simulink model "BlueROV2_Exp_Simu_NIF"  (R2023b)
settings: Solver=FixedStepAuto  StartTime=0.0  StopTime=120  FixedStep=dt  RelTol=1e-3
values from neighbouring files (symbols this model uses):
  Af = diag(ti)    [RM_param_AGF.m]
  Ballast_Force = Ballast_Compute(Ballast_Config)    [Integrate.m]    (also in init.m = Ballast_Term(Ballast_Config); init_NIF.m = [0; 0; Ballast_Term; 0]; init_NIF2.m = [0; 0; Ballast_Term; 0]; init_ODE.m)
  dt = 0.1    [Integrate.m]    (also in init.m; init_NIF.m; init_NIF2.m; init_ODE.m)
  Gamma = diag(omega_is)    [RM_param_AGF.m]
  Kd = [155; 355; 8985; 1205; 1205; 1]    [Integrate.m]    (also in init.m = [1; 1; 1; 1; 1; 1]; init_NIF.m; init_NIF2.m; init_ODE.m)
  Ki = [45; 45; 10; 96; 96; 1]    [Integrate.m]    (also in init.m = [1; 1; 1; 1; 1; 1]; init_NIF.m; init_NIF2.m; init_ODE.m)
  Kp = [255; 545; 7095; 2420; 2375; 1]    [Integrate.m]    (also in init.m = [1; 1; 1; 1; 1; 1]; init_NIF.m; init_NIF2.m; init_ODE.m)
  lower_limit = -upper_limit    (= -30)    [Integrate.m]    (also in init.m; init_NIF.m; init_NIF2.m; init_ODE.m)
  Omega = diag(2*omega_is.*zeta_is)    [RM_param_AGF.m]
  Param = BlueROV2_param()    [Integrate.m]    (also in init.m; init_NIF.m; init_NIF2.m; init_ODE.m)
  T_alloc = Thrust_Allocation()    [Integrate.m]    (also in init_NIF.m; init_NIF2.m; init_ODE.m; init_ballast_checking.m)
  T_alloc_ps = pinv(T_alloc' * T_alloc + lambda * eye(size(T_alloc, 2))) * T_alloc'    [Integrate.m]    (also in init_NIF.m; init_NIF2.m; init_ODE.m; init_ballast_checking.m)
  thrust_rate = 5    [Integrate.m]    (also in init.m; init_NIF.m; init_NIF2.m; init_ODE.m)
  upper_limit = 30    [Integrate.m]    (also in init.m; init_NIF.m; init_NIF2.m; init_ODE.m)
undefined symbols (not defined in the file or in its folder): model_val, Phi_ref, Psi_ref, resampled_time, Theta_ref, time_stamps_phi, time_stamps_psi, time_stamps_theta, time_stamps_x, time_stamps_y, time_stamps_z, time_val, X_ref, Y_ref, Z_ref
(part 1 of 2)
settings Model: Creator=goks  LastModifiedBy=HP

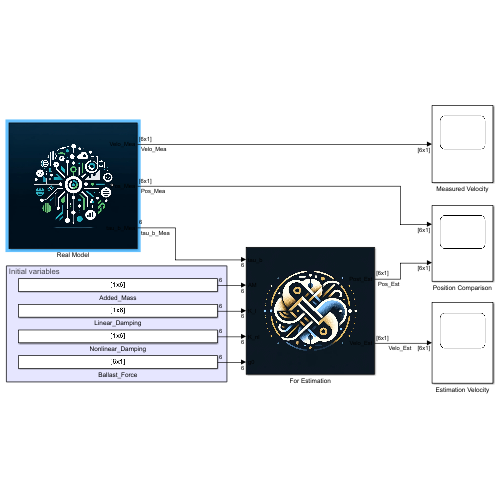
[thumbnail: Simulink's stored preview of the top-level diagram]
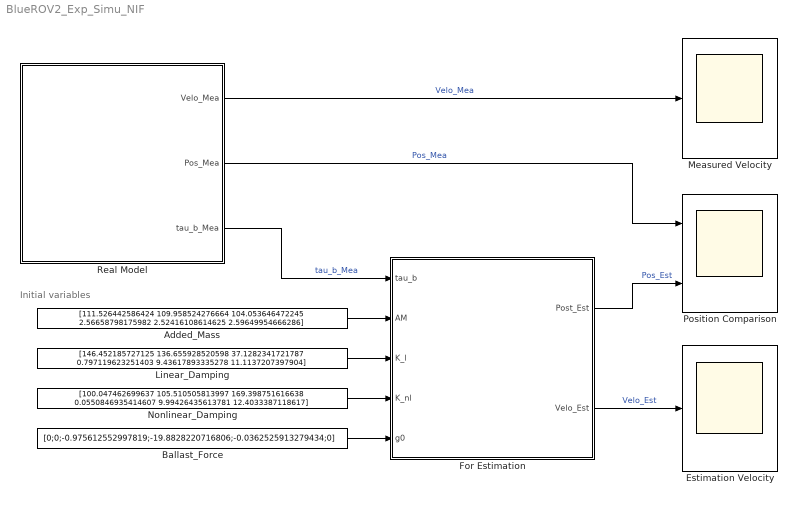
== system BlueROV2_Exp_Simu_NIF ==
  note: Initial variables
  Added_Mass : Constant  Value=[111.526442586424 109.958524276664 104.053646472245 2.56658798175982 2.52416108614625 2.59649954666286]
  Ballast_Force : Constant  Value=[0;0;-0.975612552997819;-19.8828220716806;-0.0362525913279434;0]
  Estimation Velocity : Scope
  For Estimation : Subsystem
      mask Display: image('estimated.jpg');
  Linear_Damping : Constant  Value=[146.452185727125 136.655928520598 37.1282341721787 0.797119623251403 9.43617893335278 11.1137207397904]
  Measured Velocity : Scope
  Nonlinear_Damping : Constant  Value=[100.047462699637 105.510505813997 169.398751616638 0.0550846935414607 9.99426435613781 12.4033387118617]
  Position Comparison : Scope  NumInputPorts=2
  Real Model : Subsystem
      mask Display: image('measured.jpg');
  wires:
  Real Model/1(Velo_Mea) -> Measured Velocity/1  "Velo_Mea"
  For Estimation/2(Velo_Est) -> Estimation Velocity/1  "Velo_Est"
  Added_Mass/1 -> For Estimation/2(AM)
  Linear_Damping/1 -> For Estimation/3(K_l)
  Nonlinear_Damping/1 -> For Estimation/4(K_nl)
  Real Model/2(Pos_Mea) -> Position Comparison/1  "Pos_Mea"
  For Estimation/1(Post_Est) -> Position Comparison/2  "Pos_Est"
  Real Model/3(tau_b_Mea) -> For Estimation/1(tau_b)  "tau_b_Mea"
  Ballast_Force/1 -> For Estimation/5(g0)

== system BlueROV2_Exp_Simu_NIF/For Estimation ==
  note: NIF Input
  tau_b : Inport
  AM : Inport  Port=2
  K_l : Inport  Port=3
  K_nl : Inport  Port=4
  g0 : Inport  Port=5
  BlueROV2 : Subsystem
      mask DialogControl DescTextVar Prompt: %<BlueROV2>
      mask Display: image('heavy-bluerov.jpg');
  Post_Est : Outport
  Velo_Est : Outport  Port=2
  tag scope: AM_Est=global, K_l_Est=global, K_nl_Est=global, g0_Est=global
  wires:
  tau_b/1 -> BlueROV2/1(tau_b)  "tau_b"
  AM/1 -> [AM_Est]
  K_l/1 -> [K_l_Est]
  K_nl/1 -> [K_nl_Est]
  g0/1 -> [g0_Est]
  BlueROV2/1(eta) -> Post_Est/1  "eta_n"
  BlueROV2/2(nu) -> Velo_Est/1  "nu_b"

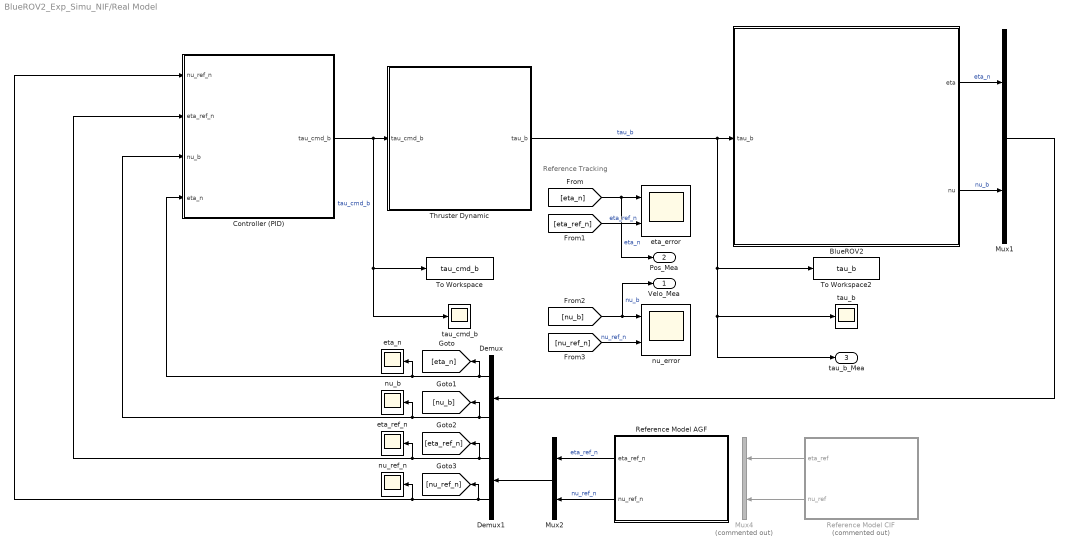
== system BlueROV2_Exp_Simu_NIF/Real Model ==
  note: Reference Tracking
  BlueROV2 : Subsystem
      mask DialogControl DescTextVar Prompt: %<BlueROV2>
      mask Display: image('heavy-bluerov.jpg');
  Controller (PID) : Subsystem
      mask Display: image('pid.jpeg');
  Demux : Demux  Outputs=2
  Demux1 : Demux  Outputs=2
  Mux1 : Mux  Inputs=2
  Mux2 : Mux  Inputs=2
  Mux4 : Mux  Commented=on  Inputs=2
  Reference Model AGF : Subsystem
      mask Display: image('ref_traj_img.png');
  Reference Model CIF : Subsystem  Commented=on
  Thruster Dynamic : Subsystem
      mask Display: image('blueROV2_heavy_config.png');
  To Workspace : ToWorkspace  VariableName=tau_cmd_b  SampleTime=-1
  To Workspace2 : ToWorkspace  VariableName=tau_b  SampleTime=-1
  eta_error : Scope  NumInputPorts=2
  eta_n : Scope
  eta_ref_n : Scope
  nu_b : Scope
  nu_error : Scope  NumInputPorts=2
  nu_ref_n : Scope
  tau_b : Scope
  tau_cmd_b : Scope
  Velo_Mea : Outport
  Pos_Mea : Outport  Port=2
  tau_b_Mea : Outport  Port=3
  wires:
  BlueROV2/1(eta) -> Mux1/1  "eta_n"
  Reference Model CIF/1(eta_ref) -> Mux4/1
  Demux/1 -> Controller (PID)/4(eta_n), eta_n/1, [eta_n]
  Controller (PID)/1(tau_cmd_b) -> tau_cmd_b/1, To Workspace/1, Thruster Dynamic/1(tau_cmd_b)  "tau_cmd_b"
  Reference Model CIF/2(nu_ref) -> Mux4/2
  Demux/2 -> Controller (PID)/3(nu_b), nu_b/1, [nu_b]
  Thruster Dynamic/1(tau_b) -> tau_b_Mea/1, tau_b/1, To Workspace2/1, BlueROV2/1(tau_b)  "tau_b"
  Demux1/2 -> Controller (PID)/1(nu_ref_n), nu_ref_n/1, [nu_ref_n]
  Reference Model AGF/1(eta_ref_n) -> Mux2/1  "eta_ref_n"
  BlueROV2/2(nu) -> Mux1/2  "nu_b"
  Mux2/1 -> Demux1/1
  Mux1/1 -> Demux/1
  Demux1/1 -> Controller (PID)/2(eta_ref_n), eta_ref_n/1, [eta_ref_n]
  Reference Model AGF/2(nu_ref_n) -> Mux2/2  "nu_ref_n"
  [eta_ref_n] -> eta_error/2  "eta_ref_n"
  [eta_n] -> Pos_Mea/1, eta_error/1  "eta_n"
  [nu_ref_n] -> nu_error/2  "nu_ref_n"
  [nu_b] -> Velo_Mea/1, nu_error/1  "nu_b"

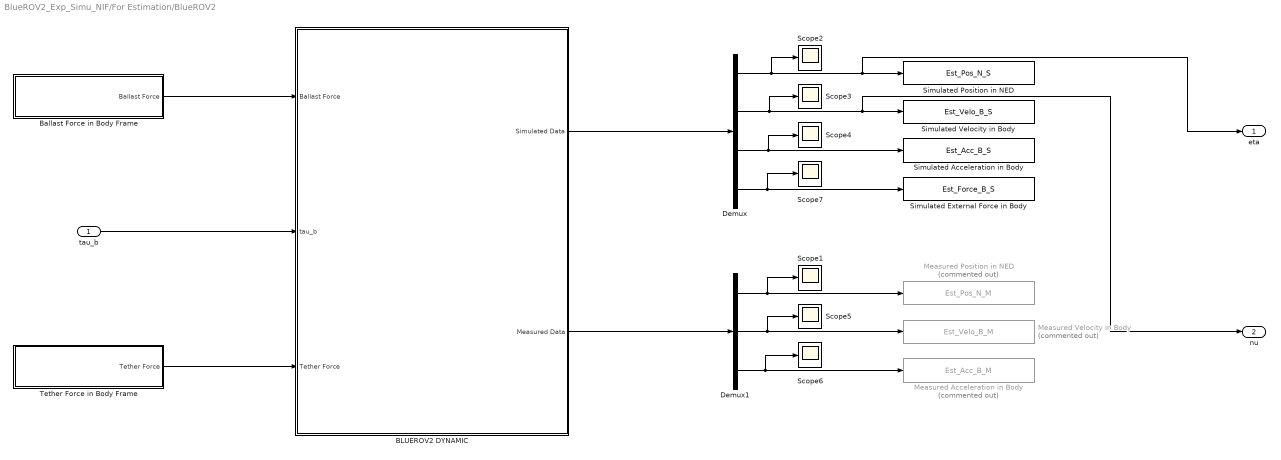
== system BlueROV2_Exp_Simu_NIF/For Estimation/BlueROV2 ==
  tau_b : Inport
  BLUEROV2 DYNAMIC : Subsystem
  Ballast Force in Body Frame : Subsystem
  Demux : Demux
  Demux1 : Demux  Outputs=3
  Measured Acceleration in Body : ToWorkspace  Commented=on  VariableName=Est_Acc_B_M  SampleTime=-1
  Measured Position in NED : ToWorkspace  Commented=on  VariableName=Est_Pos_N_M  SampleTime=-1
  Measured Velocity in Body : ToWorkspace  Commented=on  VariableName=Est_Velo_B_M  SampleTime=-1
  Scope{1..7} (7 alike) : Scope
  Simulated Acceleration in Body : ToWorkspace  VariableName=Est_Acc_B_S  SampleTime=-1
  Simulated External Force in Body : ToWorkspace  VariableName=Est_Force_B_S  SampleTime=-1
  Simulated Position in NED : ToWorkspace  VariableName=Est_Pos_N_S  SampleTime=-1
  Simulated Velocity in Body : ToWorkspace  VariableName=Est_Velo_B_S  SampleTime=-1
  Tether Force in Body Frame : Subsystem
  eta : Outport
  nu : Outport  Port=2
  wires:
  Tether Force in Body Frame/1(Tether Force) -> BLUEROV2 DYNAMIC/3(Tether Force)
  Demux/2 -> nu/1, Simulated Velocity in Body/1, Scope3/1
  BLUEROV2 DYNAMIC/1(Simulated Data) -> Demux/1
  Demux1/1 -> Measured Position in NED/1, Scope1/1
  BLUEROV2 DYNAMIC/2(Measured Data) -> Demux1/1
  Ballast Force in Body Frame/1(Ballast Force) -> BLUEROV2 DYNAMIC/1(Ballast Force)
  Demux/1 -> eta/1, Simulated Position in NED/1, Scope2/1
  Demux/3 -> Simulated Acceleration in Body/1, Scope4/1
  Demux1/2 -> Measured Velocity in Body/1, Scope5/1
  Demux1/3 -> Scope6/1, Measured Acceleration in Body/1
  Demux/4 -> Scope7/1, Simulated External Force in Body/1
  tau_b/1 -> BLUEROV2 DYNAMIC/2(tau_b)

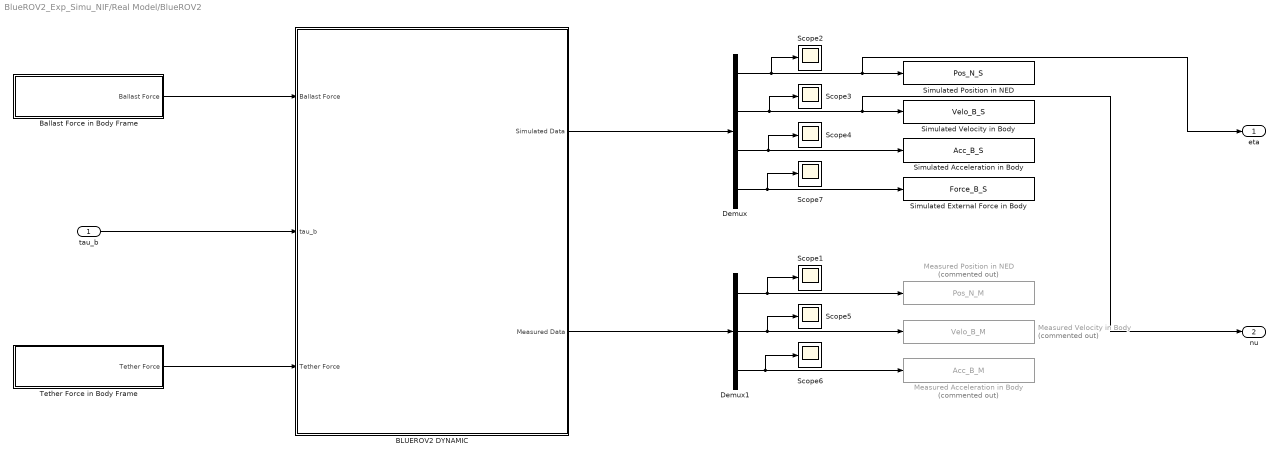
== system BlueROV2_Exp_Simu_NIF/Real Model/BlueROV2 ==
  tau_b : Inport
  BLUEROV2 DYNAMIC : Subsystem
  Ballast Force in Body Frame : Subsystem
  Demux : Demux
  Demux1 : Demux  Outputs=3
  Measured Acceleration in Body : ToWorkspace  Commented=on  VariableName=Acc_B_M  SampleTime=-1
  Measured Position in NED : ToWorkspace  Commented=on  VariableName=Pos_N_M  SampleTime=-1
  Measured Velocity in Body : ToWorkspace  Commented=on  VariableName=Velo_B_M  SampleTime=-1
  Scope{1..7} (7 alike) : Scope
  Simulated Acceleration in Body : ToWorkspace  VariableName=Acc_B_S  SampleTime=-1
  Simulated External Force in Body : ToWorkspace  VariableName=Force_B_S  SampleTime=-1
  Simulated Position in NED : ToWorkspace  VariableName=Pos_N_S  SampleTime=-1
  Simulated Velocity in Body : ToWorkspace  VariableName=Velo_B_S  SampleTime=-1
  Tether Force in Body Frame : Subsystem
  eta : Outport
  nu : Outport  Port=2
  wires:
  Tether Force in Body Frame/1(Tether Force) -> BLUEROV2 DYNAMIC/3(Tether Force)
  Demux/2 -> nu/1, Simulated Velocity in Body/1, Scope3/1
  BLUEROV2 DYNAMIC/1(Simulated Data) -> Demux/1
  Demux1/1 -> Measured Position in NED/1, Scope1/1
  BLUEROV2 DYNAMIC/2(Measured Data) -> Demux1/1
  Ballast Force in Body Frame/1(Ballast Force) -> BLUEROV2 DYNAMIC/1(Ballast Force)
  Demux/1 -> eta/1, Simulated Position in NED/1, Scope2/1
  Demux/3 -> Simulated Acceleration in Body/1, Scope4/1
  Demux1/2 -> Measured Velocity in Body/1, Scope5/1
  Demux1/3 -> Scope6/1, Measured Acceleration in Body/1
  Demux/4 -> Scope7/1, Simulated External Force in Body/1
  tau_b/1 -> BLUEROV2 DYNAMIC/2(tau_b)

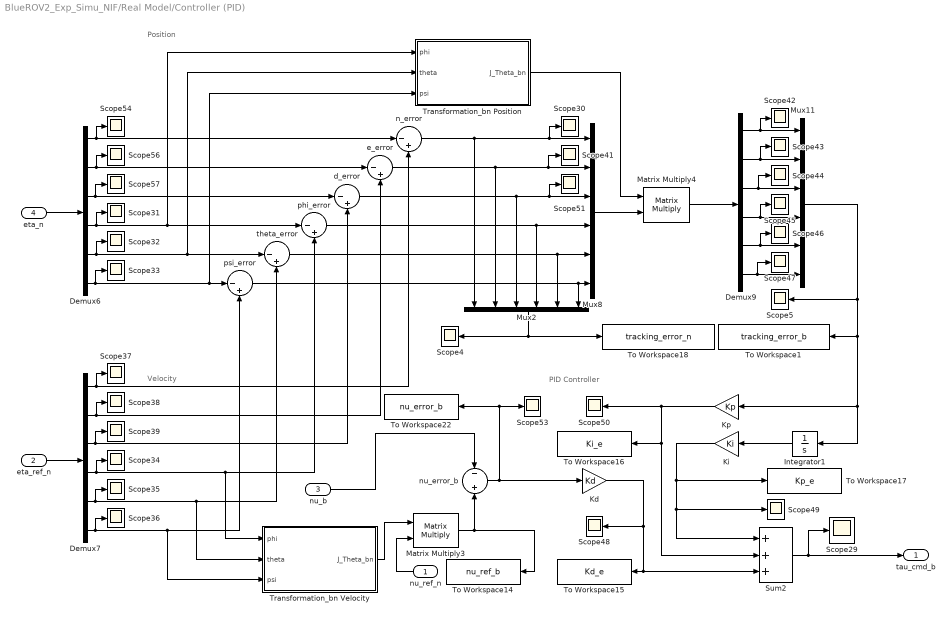
== system BlueROV2_Exp_Simu_NIF/Real Model/Controller (PID) ==
  note: Velocity
  note: PID Controller
  note: Position
  nu_ref_n : Inport
  eta_ref_n : Inport  Port=2
  nu_b : Inport  Port=3
  eta_n : Inport  Port=4
  Demux6 : Demux  Outputs=6
  Demux7 : Demux  Outputs=6
  Demux9 : Demux  Outputs=6
  Integrator1 : Integrator
  Kd : Gain  Gain=Kd
  Ki : Gain  Gain=Ki
  Kp : Gain  Gain=Kp
  Matrix Multiply3 : Product  Multiplication=Matrix(*)
  Matrix Multiply4 : Product  Multiplication=Matrix(*)
  Mux11 : Mux  Inputs=6
  Mux2 : Mux  Inputs=6
  Mux8 : Mux  Inputs=6
  Scope{4..5,29..39,41..51,53..54,56..57} (28 alike) : Scope
  Sum2 : Sum  Inputs=+++
  To Workspace1 : ToWorkspace  VariableName=tracking_error_b  SampleTime=-1
  To Workspace14 : ToWorkspace  VariableName=nu_ref_b  SampleTime=-1
  To Workspace15 : ToWorkspace  VariableName=Kd_e  SampleTime=-1
  To Workspace16 : ToWorkspace  VariableName=Ki_e  SampleTime=-1
  To Workspace17 : ToWorkspace  VariableName=Kp_e  SampleTime=-1
  To Workspace18 : ToWorkspace  VariableName=tracking_error_n  SampleTime=-1
  To Workspace22 : ToWorkspace  VariableName=nu_error_b  SampleTime=-1
  Transformation_bn Position : MATLAB Function  TreatAsAtomicUnit=on
  Transformation_bn Velocity : MATLAB Function  TreatAsAtomicUnit=on
  d_error : Sum  Inputs=|-+
  e_error : Sum  Inputs=|-+
  n_error : Sum  Inputs=|-+
  nu_error_b : Sum  Inputs=-|+
  phi_error : Sum  Inputs=|-+
  psi_error : Sum  Inputs=|-+
  theta_error : Sum  Inputs=|-+
  tau_cmd_b : Outport
  wires:
  nu_ref_n/1 -> Matrix Multiply3/2
  Demux6/5 -> theta_error/1, Transformation_bn Position/2(theta), Scope32/1
  Sum2/1 -> Scope29/1, tau_cmd_b/1
  Matrix Multiply4/1 -> Demux9/1
  Transformation_bn Velocity/1(J_Theta_bn) -> Matrix Multiply3/1
  n_error/1 -> Scope30/1, Mux8/1, Mux2/1
  Matrix Multiply3/1 -> To Workspace14/1, nu_error_b/2
  Mux2/1 -> Scope4/1, To Workspace18/1
  Demux9/2 -> Scope43/1, Mux11/2
  Demux7/1 -> Scope37/1, n_error/2
  Integrator1/1 -> Ki/1
  eta_ref_n/1 -> Demux7/1
  Mux11/1 -> Kp/1, Integrator1/1, To Workspace1/1, Scope5/1
  e_error/1 -> Scope41/1, Mux8/2, Mux2/2
  Demux9/3 -> Scope44/1, Mux11/3
  Mux8/1 -> Matrix Multiply4/2
  Demux6/2 -> Scope56/1, e_error/1
  d_error/1 -> Scope51/1, Mux8/3, Mux2/3
  Ki/1 -> Scope49/1, Sum2/1, To Workspace17/1
  Demux6/1 -> Scope54/1, n_error/1
  Kp/1 -> Scope50/1, To Workspace16/1, Sum2/2
  Kd/1 -> Sum2/3, To Workspace15/1, Scope48/1
  nu_error_b/1 -> Scope53/1, To Workspace22/1, Kd/1
  Transformation_bn Position/1(J_Theta_bn) -> Matrix Multiply4/1
  Demux7/6 -> Scope36/1, psi_error/2, Transformation_bn Velocity/3(psi)
  Demux9/1 -> Scope42/1, Mux11/1
  nu_b/1 -> nu_error_b/1
  Demux6/3 -> Scope57/1, d_error/1
  Demux7/2 -> Scope38/1, e_error/2
  phi_error/1 -> Mux8/4, Mux2/4
  theta_error/1 -> Mux8/5, Mux2/5
  psi_error/1 -> Mux8/6, Mux2/6
  Demux7/3 -> d_error/2, Scope39/1
  Demux7/5 -> Scope35/1, theta_error/2, Transformation_bn Velocity/2(theta)
  eta_n/1 -> Demux6/1
  Demux6/4 -> phi_error/1, Transformation_bn Position/1(phi), Scope31/1
  Demux6/6 -> psi_error/1, Transformation_bn Position/3(psi), Scope33/1
  Demux9/4 -> Scope45/1, Mux11/4
  Demux9/5 -> Scope46/1, Mux11/5
  Demux9/6 -> Mux11/6, Scope47/1
  Demux7/4 -> Scope34/1, Transformation_bn Velocity/1(phi), phi_error/2

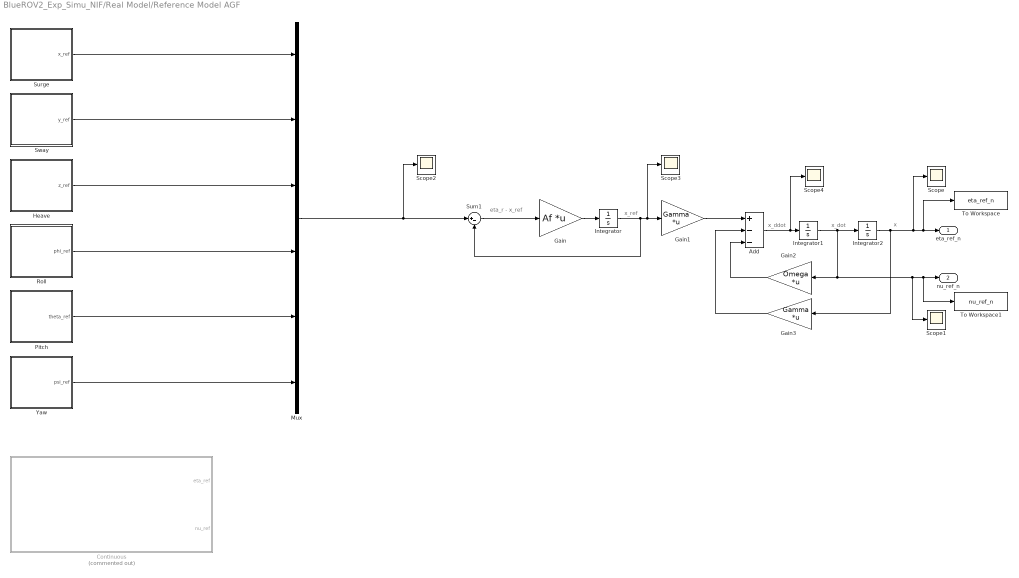
== system BlueROV2_Exp_Simu_NIF/Real Model/Reference Model AGF ==
  note: x_dot
  note: eta_r - x_ref
  note: x
  note: x_ref
  note: x_ddot
  Add : Sum  Inputs=+--
  Continuous : Subsystem  Commented=on
  Gain : Gain  Gain=Af  Multiplication=Matrix(K*u)
  Gain1 : Gain  Gain=Gamma  Multiplication=Matrix(K*u)
  Gain2 : Gain  Gain=Omega  Multiplication=Matrix(K*u)
  Gain3 : Gain  Gain=Gamma  Multiplication=Matrix(K*u)
  Heave : Subsystem
  Integrator : Integrator
  Integrator1 : Integrator
  Integrator2 : Integrator
  Mux : Mux  Inputs=6
  Pitch : Subsystem
  Roll : Subsystem
  Scope{,1..4} (5 alike) : Scope
  Sum1 : Sum  Inputs=|+-
  Surge : Subsystem
  Sway : Subsystem
  To Workspace : ToWorkspace  VariableName=eta_ref_n  SampleTime=-1
  To Workspace1 : ToWorkspace  VariableName=nu_ref_n  SampleTime=-1
  Yaw : Subsystem
  eta_ref_n : Outport
  nu_ref_n : Outport  Port=2
  wires:
  Surge/1(x_ref) -> Mux/1
  Heave/1(z_ref) -> Mux/3
  Pitch/1(theta_ref) -> Mux/5
  Yaw/1(psi_ref) -> Mux/6
  Sway/1(y_ref) -> Mux/2
  Roll/1(phi_ref) -> Mux/4
  Gain1/1 -> Add/1
  Gain/1 -> Integrator/1
  Sum1/1 -> Gain/1
  Integrator1/1 -> Integrator2/1, To Workspace1/1, nu_ref_n/1, Scope1/1, Gain2/1
  Gain3/1 -> Add/2
  Integrator2/1 -> To Workspace/1, eta_ref_n/1, Scope/1, Gain3/1
  Gain2/1 -> Add/3
  Mux/1 -> Scope2/1, Sum1/1
  Integrator/1 -> Scope3/1, Gain1/1, Sum1/2
  Add/1 -> Scope4/1, Integrator1/1

== system BlueROV2_Exp_Simu_NIF/Real Model/Reference Model CIF ==
  Heave : Subsystem
  Mux : Mux  Inputs=6
  Mux1 : Mux  Inputs=6
  Pitch : Subsystem
  Roll : Subsystem
  Scope : Scope
  Scope1 : Scope
  Surge : Subsystem
  Sway : Subsystem
  Yaw : Subsystem
  eta_ref : Outport
  nu_ref : Outport  Port=2
  wires:
  Surge/1(x_ref) -> Mux/1
  Surge/2(u_ref) -> Mux1/1
  Sway/2(v_ref) -> Mux1/2
  Heave/2(w_ref) -> Mux1/3
  Pitch/2(q_ref) -> Mux1/4
  Yaw/2(r_ref) -> Mux1/6
  Roll/2(p_ref) -> Mux1/5
  Heave/1(z_ref) -> Mux/3
  Pitch/1(theta_ref) -> Mux/5
  Yaw/1(psi_ref) -> Mux/6
  Sway/1(y_ref) -> Mux/2
  Roll/1(phi_ref) -> Mux/4
  Mux/1 -> Scope/1, eta_ref/1
  Mux1/1 -> Scope1/1, nu_ref/1

== system BlueROV2_Exp_Simu_NIF/Real Model/Thruster Dynamic ==
  tau_cmd_b : Inport
  Gain : Gain  Gain=T_alloc_ps  Multiplication=Matrix(K*u) (u vector)
  Gain1 : Gain  Gain=T_alloc  Multiplication=Matrix(K*u) (u vector)
  Manual Switch : ManualSwitch
  Saturation and Dynamics : Subsystem
      mask Display: image('t200-img.jpg');
  Scope : Scope
  Scope1 : Scope
  tau_b : Outport
  wires:
  Manual Switch/1 -> Gain1/1
  tau_cmd_b/1 -> Gain/1
  Gain/1 -> Scope/1, Saturation and Dynamics/1(Commanded Thrust), Manual Switch/2
  Gain1/1 -> tau_b/1
  Saturation and Dynamics/1(Actual Thrust) -> Scope1/1, Manual Switch/1

== system BlueROV2_Exp_Simu_NIF/For Estimation/BlueROV2/BLUEROV2 DYNAMIC ==
  Ballast Force : Inport
  tau_b : Inport  Port=2
  Tether Force : Inport  Port=3
  Manual Switch : ManualSwitch
  Mux : Mux
  Mux1 : Mux  Inputs=3
  ROV_SYSTEM : Subsystem
  SIMULATED - MEASURED w. NOISE : Subsystem
  To Workspace2 : ToWorkspace  VariableName=Est_BF  SampleTime=-1
  To Workspace3 : ToWorkspace  VariableName=Est_TF  SampleTime=-1
  To Workspace4 : ToWorkspace  VariableName=Est_TtF  SampleTime=-1
  Simulated Data : Outport
  Measured Data : Outport  Port=2
  wires:
  ROV_SYSTEM/1(Position and Orientation in NED (m and rad)) -> Mux/1
  ROV_SYSTEM/2(Velocity in Body (m/s and rad/s)) -> Mux/2
  ROV_SYSTEM/3(Acceleration in B (m/s² and rad/s²)) -> Mux/3
  ROV_SYSTEM/4(Force (N)) -> Mux/4
  SIMULATED - MEASURED w. NOISE/2(Measured Velocity in Body) -> Mux1/2
  SIMULATED - MEASURED w. NOISE/1(Measured Position and Orientation in NED) -> Mux1/1
  SIMULATED - MEASURED w. NOISE/3(Measured Acceleration in Body) -> Mux1/3
  Mux/1 -> SIMULATED - MEASURED w. NOISE/1(Simulated Data), Manual Switch/1, Simulated Data/1  "SIMULATED - MEASURED - wo. NOISE"
  Manual Switch/1 -> Measured Data/1
  Mux1/1 -> Manual Switch/2
  Ballast Force/1 -> ROV_SYSTEM/1(Ballast Force), To Workspace2/1
  tau_b/1 -> ROV_SYSTEM/2(tau_b), To Workspace3/1
  Tether Force/1 -> To Workspace4/1, ROV_SYSTEM/3(Tether Force)

== system BlueROV2_Exp_Simu_NIF/For Estimation/BlueROV2/Ballast Force in Body Frame ==
  Ballast : Step  Time=0  Before=[0;0;-0.975612552997819;-19.8828220716806;-0.0362525913279434;0]  After=[0;0;-0.975612552997819;-19.8828220716806;-0.0362525913279434;0]  SampleTime=0
  Scope : Scope
  Ballast Force : Outport
  wires:
  Ballast/1 -> Scope/1, Ballast Force/1

== system BlueROV2_Exp_Simu_NIF/For Estimation/BlueROV2/Tether Force in Body Frame ==
  Scope : Scope
  Tether : Step  Before=zeros(6,1)  After=zeros(6,1)  SampleTime=0
  Tether Force : Outport
  wires:
  Tether/1 -> Scope/1, Tether Force/1

== system BlueROV2_Exp_Simu_NIF/Real Model/BlueROV2/BLUEROV2 DYNAMIC ==
  Ballast Force : Inport
  tau_b : Inport  Port=2
  Tether Force : Inport  Port=3
  Manual Switch : ManualSwitch
  Mux : Mux
  Mux1 : Mux  Inputs=3
  ROV_SYSTEM : Subsystem
  SIMULATED - MEASURED w. NOISE : Subsystem
  To Workspace2 : ToWorkspace  VariableName=BF  SampleTime=-1
  To Workspace3 : ToWorkspace  VariableName=TF  SampleTime=-1
  To Workspace4 : ToWorkspace  VariableName=TtF  SampleTime=-1
  Simulated Data : Outport
  Measured Data : Outport  Port=2
  wires:
  ROV_SYSTEM/1(Position and Orientation in NED (m and rad)) -> Mux/1
  ROV_SYSTEM/2(Velocity in Body (m/s and rad/s)) -> Mux/2
  ROV_SYSTEM/3(Acceleration in B (m/s² and rad/s²)) -> Mux/3
  ROV_SYSTEM/4(Force (N)) -> Mux/4
  SIMULATED - MEASURED w. NOISE/2(Measured Velocity in Body) -> Mux1/2
  SIMULATED - MEASURED w. NOISE/1(Measured Position and Orientation in NED) -> Mux1/1
  SIMULATED - MEASURED w. NOISE/3(Measured Acceleration in Body) -> Mux1/3
  Mux/1 -> SIMULATED - MEASURED w. NOISE/1(Simulated Data), Manual Switch/1, Simulated Data/1  "SIMULATED - MEASURED - wo. NOISE"
  Manual Switch/1 -> Measured Data/1
  Mux1/1 -> Manual Switch/2
  Ballast Force/1 -> ROV_SYSTEM/1(Ballast Force), To Workspace2/1
  tau_b/1 -> ROV_SYSTEM/2(tau_b), To Workspace3/1
  Tether Force/1 -> To Workspace4/1, ROV_SYSTEM/3(Tether Force)

== system BlueROV2_Exp_Simu_NIF/Real Model/BlueROV2/Ballast Force in Body Frame ==
  Ballast : Step  Time=0  Before=Ballast_Force  After=Ballast_Force  SampleTime=0
  Scope : Scope
  Ballast Force : Outport
  wires:
  Ballast/1 -> Scope/1, Ballast Force/1

== system BlueROV2_Exp_Simu_NIF/Real Model/BlueROV2/Tether Force in Body Frame ==
  Scope : Scope
  Tether : Step  Before=zeros(6,1)  After=zeros(6,1)  SampleTime=0
  Tether Force : Outport
  wires:
  Tether/1 -> Scope/1, Tether Force/1

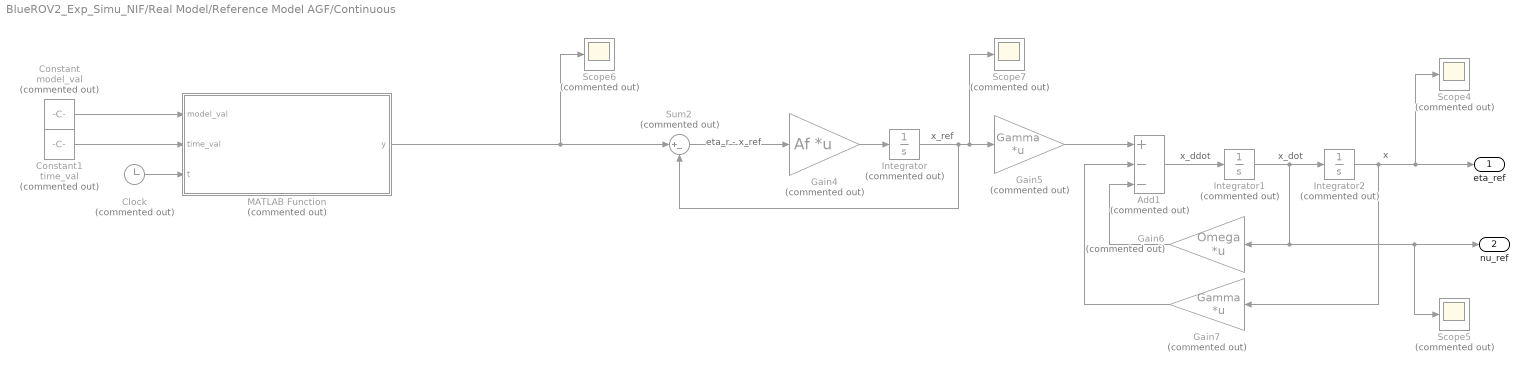
== system BlueROV2_Exp_Simu_NIF/Real Model/Reference Model AGF/Continuous ==
  note: x_dot
  note: x_ddot
  note: x
  note: eta_r - x_ref
  note: x_ref
  Add1 : Sum  Commented=on  Inputs=+--
  Clock : Clock  Commented=on
  Constant : Constant  Commented=on  Value=model_val
  Constant1 : Constant  Commented=on  Value=time_val
  Gain4 : Gain  Commented=on  Gain=Af  Multiplication=Matrix(K*u)
  Gain5 : Gain  Commented=on  Gain=Gamma  Multiplication=Matrix(K*u)
  Gain6 : Gain  Commented=on  Gain=Omega  Multiplication=Matrix(K*u)
  Gain7 : Gain  Commented=on  Gain=Gamma  Multiplication=Matrix(K*u)
  Integrator : Integrator  Commented=on
  Integrator1 : Integrator  Commented=on
  Integrator2 : Integrator  Commented=on
  MATLAB Function : MATLAB Function  Commented=on  TreatAsAtomicUnit=on
  Scope{4..7} (4 alike) : Scope  Commented=on
  Sum2 : Sum  Commented=on  Inputs=|+-
  eta_ref : Outport
  nu_ref : Outport  Port=2
  wires:
  Gain7/1 -> Add1/2
  Clock/1 -> MATLAB Function/3(t)
  Gain6/1 -> Add1/3
  Integrator/1 -> Scope7/1, Gain5/1, Sum2/2
  Add1/1 -> Integrator1/1
  Constant/1 -> MATLAB Function/1(model_val)
  Gain4/1 -> Integrator/1
  Gain5/1 -> Add1/1
  Integrator1/1 -> Integrator2/1, nu_ref/1, Scope5/1, Gain6/1
  MATLAB Function/1(y) -> Scope6/1, Sum2/1
  Sum2/1 -> Gain4/1
  Integrator2/1 -> eta_ref/1, Scope4/1, Gain7/1
  Constant1/1 -> MATLAB Function/2(time_val)

== system BlueROV2_Exp_Simu_NIF/Real Model/Reference Model AGF/Heave ==
  Clock1 : Clock
  Constant2 : Constant  Value=Z_ref
  Constant3 : Constant  Value=time_stamps_z
  MATLAB Function1 : MATLAB Function  TreatAsAtomicUnit=on
  z_ref : Outport
  wires:
  Constant3/1 -> MATLAB Function1/2(time_stamps)
  MATLAB Function1/1(ref) -> z_ref/1
  Clock1/1 -> MATLAB Function1/3(t)
  Constant2/1 -> MATLAB Function1/1(val_checkpoints)

== system BlueROV2_Exp_Simu_NIF/Real Model/Reference Model AGF/Pitch ==
  Clock1 : Clock
  Constant2 : Constant  Value=Theta_ref
  Constant3 : Constant  Value=time_stamps_theta
  MATLAB Function1 : MATLAB Function  TreatAsAtomicUnit=on
  theta_ref : Outport
  wires:
  Constant3/1 -> MATLAB Function1/2(time_stamps)
  MATLAB Function1/1(ref) -> theta_ref/1
  Clock1/1 -> MATLAB Function1/3(t)
  Constant2/1 -> MATLAB Function1/1(val_checkpoints)

== system BlueROV2_Exp_Simu_NIF/Real Model/Reference Model AGF/Roll ==
  Clock1 : Clock
  Constant2 : Constant  Value=Phi_ref
  Constant3 : Constant  Value=time_stamps_phi
  MATLAB Function1 : MATLAB Function  TreatAsAtomicUnit=on
  phi_ref : Outport
  wires:
  Constant3/1 -> MATLAB Function1/2(time_stamps)
  MATLAB Function1/1(ref) -> phi_ref/1
  Clock1/1 -> MATLAB Function1/3(t)
  Constant2/1 -> MATLAB Function1/1(val_checkpoints)

== system BlueROV2_Exp_Simu_NIF/Real Model/Reference Model AGF/Surge ==
  Clock1 : Clock
  Constant2 : Constant  Value=X_ref
  Constant3 : Constant  Value=time_stamps_x
  MATLAB Function1 : MATLAB Function  TreatAsAtomicUnit=on
  x_ref : Outport
  wires:
  MATLAB Function1/1(ref) -> x_ref/1
  Clock1/1 -> MATLAB Function1/3(t)
  Constant2/1 -> MATLAB Function1/1(val_checkpoints)
  Constant3/1 -> MATLAB Function1/2(time_stamps)

== system BlueROV2_Exp_Simu_NIF/Real Model/Reference Model AGF/Sway ==
  Clock1 : Clock
  Constant2 : Constant  Value=Y_ref
  Constant3 : Constant  Value=time_stamps_y
  MATLAB Function1 : MATLAB Function  TreatAsAtomicUnit=on
  y_ref : Outport
  wires:
  Constant3/1 -> MATLAB Function1/2(time_stamps)
  MATLAB Function1/1(ref) -> y_ref/1
  Clock1/1 -> MATLAB Function1/3(t)
  Constant2/1 -> MATLAB Function1/1(val_checkpoints)

== system BlueROV2_Exp_Simu_NIF/Real Model/Reference Model AGF/Yaw ==
  Clock1 : Clock
  Constant2 : Constant  Value=Psi_ref
  Constant3 : Constant  Value=time_stamps_psi
  MATLAB Function1 : MATLAB Function  TreatAsAtomicUnit=on
  psi_ref : Outport
  wires:
  Constant3/1 -> MATLAB Function1/2(time_stamps)
  MATLAB Function1/1(ref) -> psi_ref/1
  Clock1/1 -> MATLAB Function1/3(t)
  Constant2/1 -> MATLAB Function1/1(val_checkpoints)

== system BlueROV2_Exp_Simu_NIF/Real Model/Reference Model CIF/Heave ==
  Clock : Clock
  Constant : Constant  Value=Z_ref
  Constant1 : Constant  Value=resampled_time
  Derivative : Derivative
  First Order Hold : FirstOrderHold  ErrorTolerance=inf  AllowContinuousInput=on
  MATLAB Function : MATLAB Function  TreatAsAtomicUnit=on
  Zero-Order Hold : ZeroOrderHold  SampleTime=-1
  z_ref : Outport
  w_ref : Outport  Port=2
  wires:
  Constant/1 -> MATLAB Function/2(resampled_model)
  Constant1/1 -> MATLAB Function/3(resampled_time)
  Clock/1 -> MATLAB Function/1(t)
  Derivative/1 -> w_ref/1
  First Order Hold/1 -> Derivative/1, z_ref/1
  MATLAB Function/1(eta_ref) -> Zero-Order Hold/1
  Zero-Order Hold/1 -> First Order Hold/1

== system BlueROV2_Exp_Simu_NIF/Real Model/Reference Model CIF/Pitch ==
  Clock : Clock
  Constant : Constant  Value=Theta_ref
  Constant1 : Constant  Value=resampled_time
  Derivative : Derivative
  First Order Hold : FirstOrderHold  ErrorTolerance=inf  AllowContinuousInput=on
  MATLAB Function : MATLAB Function  TreatAsAtomicUnit=on
  Zero-Order Hold : ZeroOrderHold  SampleTime=-1
  theta_ref : Outport
  q_ref : Outport  Port=2
  wires:
  Constant/1 -> MATLAB Function/2(resampled_model)
  Constant1/1 -> MATLAB Function/3(resampled_time)
  Clock/1 -> MATLAB Function/1(t)
  Derivative/1 -> q_ref/1
  First Order Hold/1 -> Derivative/1, theta_ref/1
  MATLAB Function/1(eta_ref) -> Zero-Order Hold/1
  Zero-Order Hold/1 -> First Order Hold/1

== system BlueROV2_Exp_Simu_NIF/Real Model/Reference Model CIF/Roll ==
  Clock : Clock
  Constant : Constant  Value=Phi_ref
  Constant1 : Constant  Value=resampled_time
  Derivative : Derivative
  First Order Hold : FirstOrderHold  ErrorTolerance=inf  AllowContinuousInput=on
  MATLAB Function : MATLAB Function  TreatAsAtomicUnit=on
  Zero-Order Hold : ZeroOrderHold  SampleTime=-1
  phi_ref : Outport
  p_ref : Outport  Port=2
  wires:
  Constant/1 -> MATLAB Function/2(resampled_model)
  Constant1/1 -> MATLAB Function/3(resampled_time)
  Clock/1 -> MATLAB Function/1(t)
  MATLAB Function/1(eta_ref) -> Zero-Order Hold/1
  Derivative/1 -> p_ref/1
  First Order Hold/1 -> Derivative/1, phi_ref/1
  Zero-Order Hold/1 -> First Order Hold/1

== system BlueROV2_Exp_Simu_NIF/Real Model/Reference Model CIF/Surge ==
  Clock : Clock
  Constant : Constant  Value=X_ref
  Constant1 : Constant  Value=resampled_time
  Derivative : Derivative
  First Order Hold : FirstOrderHold  ErrorTolerance=inf  AllowContinuousInput=on
  MATLAB Function : MATLAB Function  TreatAsAtomicUnit=on
  Zero-Order Hold : ZeroOrderHold  SampleTime=-1
  x_ref : Outport
  u_ref : Outport  Port=2
  wires:
  Constant/1 -> MATLAB Function/2(resampled_model)
  Constant1/1 -> MATLAB Function/3(resampled_time)
  Clock/1 -> MATLAB Function/1(t)
  MATLAB Function/1(eta_ref) -> Zero-Order Hold/1
  Derivative/1 -> u_ref/1
  First Order Hold/1 -> Derivative/1, x_ref/1
  Zero-Order Hold/1 -> First Order Hold/1

== system BlueROV2_Exp_Simu_NIF/Real Model/Reference Model CIF/Sway ==
  Clock : Clock
  Constant : Constant  Value=Y_ref
  Constant1 : Constant  Value=resampled_time
  Derivative : Derivative
  First Order Hold : FirstOrderHold  ErrorTolerance=inf  AllowContinuousInput=on
  MATLAB Function : MATLAB Function  TreatAsAtomicUnit=on
  Zero-Order Hold : ZeroOrderHold  SampleTime=-1
  y_ref : Outport
  v_ref : Outport  Port=2
  wires:
  Constant/1 -> MATLAB Function/2(resampled_model)
  Constant1/1 -> MATLAB Function/3(resampled_time)
  Clock/1 -> MATLAB Function/1(t)
  MATLAB Function/1(eta_ref) -> Zero-Order Hold/1
  Derivative/1 -> v_ref/1
  First Order Hold/1 -> Derivative/1, y_ref/1
  Zero-Order Hold/1 -> First Order Hold/1

== system BlueROV2_Exp_Simu_NIF/Real Model/Reference Model CIF/Yaw ==
  Clock : Clock
  Constant : Constant  Value=Psi_ref
  Constant1 : Constant  Value=resampled_time
  Derivative : Derivative
  First Order Hold : FirstOrderHold  ErrorTolerance=inf  AllowContinuousInput=on
  MATLAB Function : MATLAB Function  TreatAsAtomicUnit=on
  Zero-Order Hold : ZeroOrderHold  SampleTime=-1
  psi_ref : Outport
  r_ref : Outport  Port=2
  wires:
  Constant/1 -> MATLAB Function/2(resampled_model)
  Constant1/1 -> MATLAB Function/3(resampled_time)
  Clock/1 -> MATLAB Function/1(t)
  Derivative/1 -> r_ref/1
  First Order Hold/1 -> Derivative/1, psi_ref/1
  MATLAB Function/1(eta_ref) -> Zero-Order Hold/1
  Zero-Order Hold/1 -> First Order Hold/1

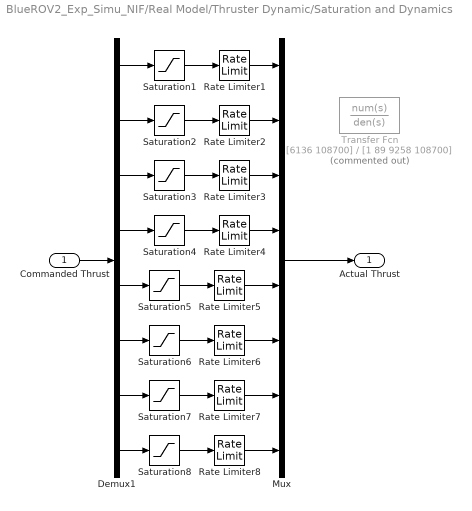
== system BlueROV2_Exp_Simu_NIF/Real Model/Thruster Dynamic/Saturation and Dynamics ==
  Commanded Thrust : Inport
  Demux1 : Demux  Outputs=8
  Mux : Mux  Inputs=8
  Rate Limiter{1..8} (8 alike) : RateLimiter  RisingSlewLimit=thrust_rate  FallingSlewLimit=-thrust_rate  SampleTimeMode=inherited
  Saturation{1..8} (8 alike) : Saturate  UpperLimit=upper_limit  LowerLimit=lower_limit
  Transfer Fcn : TransferFcn  Commented=on  Numerator=[6136 108700]  Denominator=[1 89 9258 108700]  ParameterTunability=Optimized
  Actual Thrust : Outport
  wires:
  Demux1/4 -> Saturation4/1
  Saturation2/1 -> Rate Limiter2/1
  Demux1/5 -> Saturation5/1
  Demux1/2 -> Saturation2/1
  Demux1/8 -> Saturation8/1
  Demux1/3 -> Saturation3/1
  Saturation1/1 -> Rate Limiter1/1
  Demux1/6 -> Saturation6/1
  Demux1/7 -> Saturation7/1
  Saturation8/1 -> Rate Limiter8/1
  Saturation5/1 -> Rate Limiter5/1
  Saturation3/1 -> Rate Limiter3/1
  Saturation6/1 -> Rate Limiter6/1
  Saturation7/1 -> Rate Limiter7/1
  Demux1/1 -> Saturation1/1
  Saturation4/1 -> Rate Limiter4/1
  Commanded Thrust/1 -> Demux1/1
  Mux/1 -> Actual Thrust/1
  Rate Limiter1/1 -> Mux/1
  Rate Limiter2/1 -> Mux/2
  Rate Limiter3/1 -> Mux/3
  Rate Limiter4/1 -> Mux/4
  Rate Limiter6/1 -> Mux/6
  Rate Limiter7/1 -> Mux/7
  Rate Limiter8/1 -> Mux/8
  Rate Limiter5/1 -> Mux/5

== system BlueROV2_Exp_Simu_NIF/For Estimation/BlueROV2/BLUEROV2 DYNAMIC/ROV_SYSTEM ==
  Ballast Force : Inport
  tau_b : Inport  Port=2
  Tether Force : Inport  Port=3
  DYNAMIC SOLVER : Subsystem
  Position and Orientation in NED (m and rad) : Outport
  Velocity in Body (m/s and rad/s) : Outport  Port=2
  Acceleration in B (m/s² and rad/s²) : Outport  Port=3
  Force (N) : Outport  Port=4
  wires:
  DYNAMIC SOLVER/2(Velocity in Body (m/s and rad/s)) -> Velocity in Body (m/s and rad/s)/1
  DYNAMIC SOLVER/1(Position and Orientation in NED (m and rad)) -> Position and Orientation in NED (m and rad)/1
  DYNAMIC SOLVER/3(Acceleration in B (m/s² and rad/s²)) -> Acceleration in B (m/s² and rad/s²)/1
  tau_b/1 -> DYNAMIC SOLVER/2(tau_b), Force (N)/1
  Ballast Force/1 -> DYNAMIC SOLVER/1(Ballast Force)
  Tether Force/1 -> DYNAMIC SOLVER/3(Tether Force)

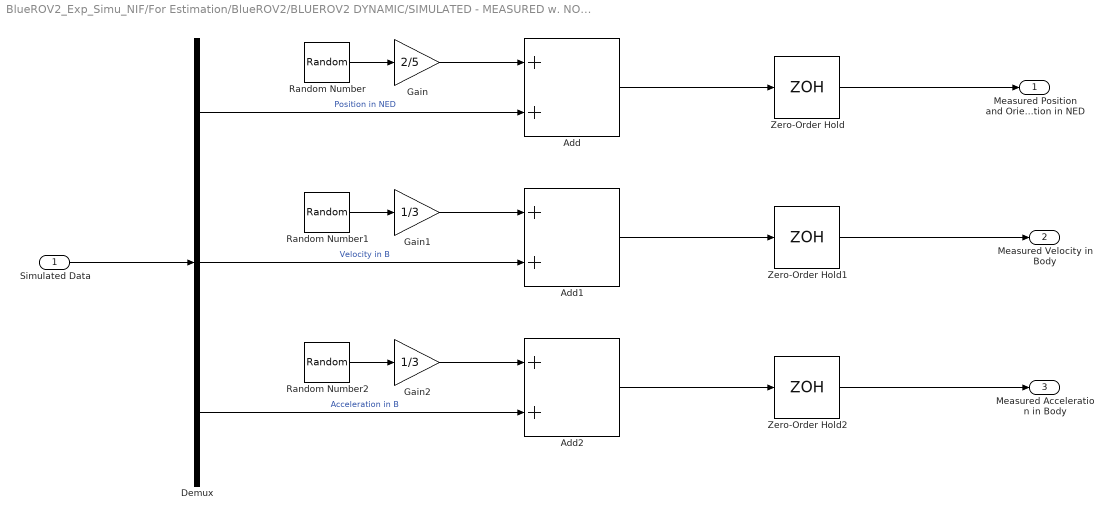
== system BlueROV2_Exp_Simu_NIF/For Estimation/BlueROV2/BLUEROV2 DYNAMIC/SIMULATED - MEASURED w. NOISE ==
  Simulated Data : Inport
  Add : Sum
  Add1 : Sum
  Add2 : Sum
  Demux : Demux  Outputs=3
  Gain : Gain  Gain=2/5
  Gain1 : Gain  Gain=1/3
  Gain2 : Gain  Gain=1/3
  Random Number : RandomNumber  Variance=0.01  SampleTime=dt
  Random Number1 : RandomNumber  Variance=0.01  SampleTime=dt
  Random Number2 : RandomNumber  Variance=0.01  SampleTime=dt
  Zero-Order Hold : ZeroOrderHold  SampleTime=-1
  Zero-Order Hold1 : ZeroOrderHold  SampleTime=-1
  Zero-Order Hold2 : ZeroOrderHold  SampleTime=-1
  Measured Position and Orientation in NED : Outport
  Measured Velocity in Body : Outport  Port=2
  Measured Acceleration in Body : Outport  Port=3
  wires:
  Simulated Data/1 -> Demux/1
  Demux/1 -> Add/2  "Position in NED"
  Random Number/1 -> Gain/1
  Gain/1 -> Add/1
  Random Number1/1 -> Gain1/1
  Demux/2 -> Add1/2  "Velocity in B"
  Gain1/1 -> Add1/1
  Random Number2/1 -> Gain2/1
  Demux/3 -> Add2/2  "Acceleration in B"
  Gain2/1 -> Add2/1
  Add/1 -> Zero-Order Hold/1
  Add1/1 -> Zero-Order Hold1/1
  Add2/1 -> Zero-Order Hold2/1
  Zero-Order Hold/1 -> Measured Position and Orientation in NED/1
  Zero-Order Hold1/1 -> Measured Velocity in Body/1
  Zero-Order Hold2/1 -> Measured Acceleration in Body/1

== system BlueROV2_Exp_Simu_NIF/Real Model/BlueROV2/BLUEROV2 DYNAMIC/ROV_SYSTEM ==
  Ballast Force : Inport
  tau_b : Inport  Port=2
  Tether Force : Inport  Port=3
  DYNAMIC SOLVER : Subsystem
  Position and Orientation in NED (m and rad) : Outport
  Velocity in Body (m/s and rad/s) : Outport  Port=2
  Acceleration in B (m/s² and rad/s²) : Outport  Port=3
  Force (N) : Outport  Port=4
  wires:
  DYNAMIC SOLVER/2(Velocity in Body (m/s and rad/s)) -> Velocity in Body (m/s and rad/s)/1
  DYNAMIC SOLVER/1(Position and Orientation in NED (m and rad)) -> Position and Orientation in NED (m and rad)/1
  DYNAMIC SOLVER/3(Acceleration in B (m/s² and rad/s²)) -> Acceleration in B (m/s² and rad/s²)/1
  tau_b/1 -> DYNAMIC SOLVER/2(tau_b), Force (N)/1
  Ballast Force/1 -> DYNAMIC SOLVER/1(Ballast Force)
  Tether Force/1 -> DYNAMIC SOLVER/3(Tether Force)

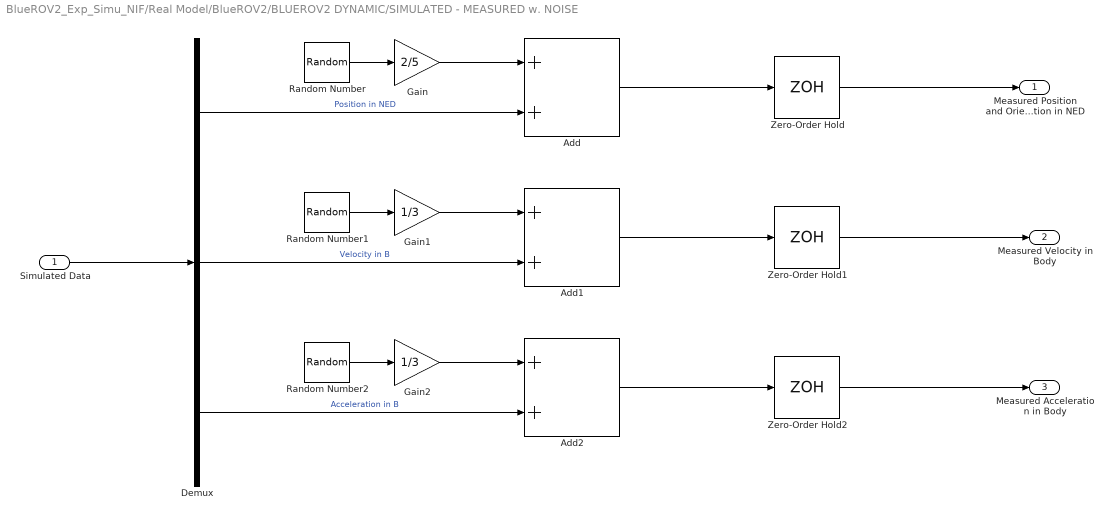
== system BlueROV2_Exp_Simu_NIF/Real Model/BlueROV2/BLUEROV2 DYNAMIC/SIMULATED - MEASURED w. NOISE ==
  Simulated Data : Inport
  Add : Sum
  Add1 : Sum
  Add2 : Sum
  Demux : Demux  Outputs=3
  Gain : Gain  Gain=2/5
  Gain1 : Gain  Gain=1/3
  Gain2 : Gain  Gain=1/3
  Random Number : RandomNumber  Variance=0.01  SampleTime=dt
  Random Number1 : RandomNumber  Variance=0.01  SampleTime=dt
  Random Number2 : RandomNumber  Variance=0.01  SampleTime=dt
  Zero-Order Hold : ZeroOrderHold  SampleTime=-1
  Zero-Order Hold1 : ZeroOrderHold  SampleTime=-1
  Zero-Order Hold2 : ZeroOrderHold  SampleTime=-1
  Measured Position and Orientation in NED : Outport
  Measured Velocity in Body : Outport  Port=2
  Measured Acceleration in Body : Outport  Port=3
  wires:
  Simulated Data/1 -> Demux/1
  Demux/1 -> Add/2  "Position in NED"
  Random Number/1 -> Gain/1
  Gain/1 -> Add/1
  Random Number1/1 -> Gain1/1
  Demux/2 -> Add1/2  "Velocity in B"
  Gain1/1 -> Add1/1
  Random Number2/1 -> Gain2/1
  Demux/3 -> Add2/2  "Acceleration in B"
  Gain2/1 -> Add2/1
  Add/1 -> Zero-Order Hold/1
  Add1/1 -> Zero-Order Hold1/1
  Add2/1 -> Zero-Order Hold2/1
  Zero-Order Hold/1 -> Measured Position and Orientation in NED/1
  Zero-Order Hold1/1 -> Measured Velocity in Body/1
  Zero-Order Hold2/1 -> Measured Acceleration in Body/1

== system BlueROV2_Exp_Simu_NIF/For Estimation/BlueROV2/BLUEROV2 DYNAMIC/ROV_SYSTEM/DYNAMIC SOLVER ==
  note: Velocity in {b} integration to position and orientation in {n}
  note: Acceleration integration to velocity in {b}
  Ballast Force : Inport
  tau_b : Inport  Port=2
  Tether Force : Inport  Port=3
  Acceleration Integrator : Integrator  InitialCondition=Param.IC.Velo
  BlueROV2_EOM : Subsystem
  Matrix Multiply : Product  Multiplication=Matrix(*)
  Rotation Matrix : MATLAB Function  TreatAsAtomicUnit=on
  Scope{,1..5} (6 alike) : Scope
  Velocity Integrator : Integrator  InitialCondition=Param.IC.Pos
  Position and Orientation in NED (m and rad) : Outport
  Velocity in Body (m/s and rad/s) : Outport  Port=2
  Acceleration in B (m/s² and rad/s²) : Outport  Port=3
  wires:
  tau_b/1 -> BlueROV2_EOM/2(tau_b), Scope/1
  Rotation Matrix/1(J_Theta_nb) -> Matrix Multiply/1
  Matrix Multiply/1 -> Velocity Integrator/1  "eta_dot_n"
  Ballast Force/1 -> Scope2/1, BlueROV2_EOM/1(Ballast Force)
  BlueROV2_EOM/1(acc_b) -> Acceleration Integrator/1, Acceleration in B (m/s² and rad/s²)/1, Scope3/1  "nu_dot_b"
  Tether Force/1 -> BlueROV2_EOM/3(Tether Force), Scope1/1
  Velocity Integrator/1 -> Rotation Matrix/1(eta_n), Position and Orientation in NED (m and rad)/1, BlueROV2_EOM/4(eta_n), Scope5/1  "eta_n"
  Acceleration Integrator/1 -> Scope4/1, BlueROV2_EOM/5(nu_b), Velocity in Body (m/s and rad/s)/1, Matrix Multiply/2  "nu_b"

== system BlueROV2_Exp_Simu_NIF/Real Model/BlueROV2/BLUEROV2 DYNAMIC/ROV_SYSTEM/DYNAMIC SOLVER ==
  note: Velocity in {b} integration to position and orientation in {n}
  note: Acceleration integration to velocity in {b}
  Ballast Force : Inport
  tau_b : Inport  Port=2
  Tether Force : Inport  Port=3
  Acceleration Integrator : Integrator  InitialCondition=Param.IC.Velo
  BlueROV2_EOM : Subsystem
  Matrix Multiply : Product  Multiplication=Matrix(*)
  Rotation Matrix : MATLAB Function  TreatAsAtomicUnit=on
  Scope{,1..5} (6 alike) : Scope
  Velocity Integrator : Integrator  InitialCondition=Param.IC.Pos
  Position and Orientation in NED (m and rad) : Outport
  Velocity in Body (m/s and rad/s) : Outport  Port=2
  Acceleration in B (m/s² and rad/s²) : Outport  Port=3
  wires:
  tau_b/1 -> BlueROV2_EOM/2(tau_b), Scope/1
  Rotation Matrix/1(J_Theta_nb) -> Matrix Multiply/1
  Matrix Multiply/1 -> Velocity Integrator/1  "eta_dot_n"
  Ballast Force/1 -> Scope2/1, BlueROV2_EOM/1(Ballast Force)
  BlueROV2_EOM/1(acc_b) -> Acceleration Integrator/1, Acceleration in B (m/s² and rad/s²)/1, Scope3/1  "nu_dot_b"
  Tether Force/1 -> BlueROV2_EOM/3(Tether Force), Scope1/1
  Velocity Integrator/1 -> Rotation Matrix/1(eta_n), Position and Orientation in NED (m and rad)/1, BlueROV2_EOM/4(eta_n), Scope5/1  "eta_n"
  Acceleration Integrator/1 -> Scope4/1, BlueROV2_EOM/5(nu_b), Velocity in Body (m/s and rad/s)/1, Matrix Multiply/2  "nu_b"

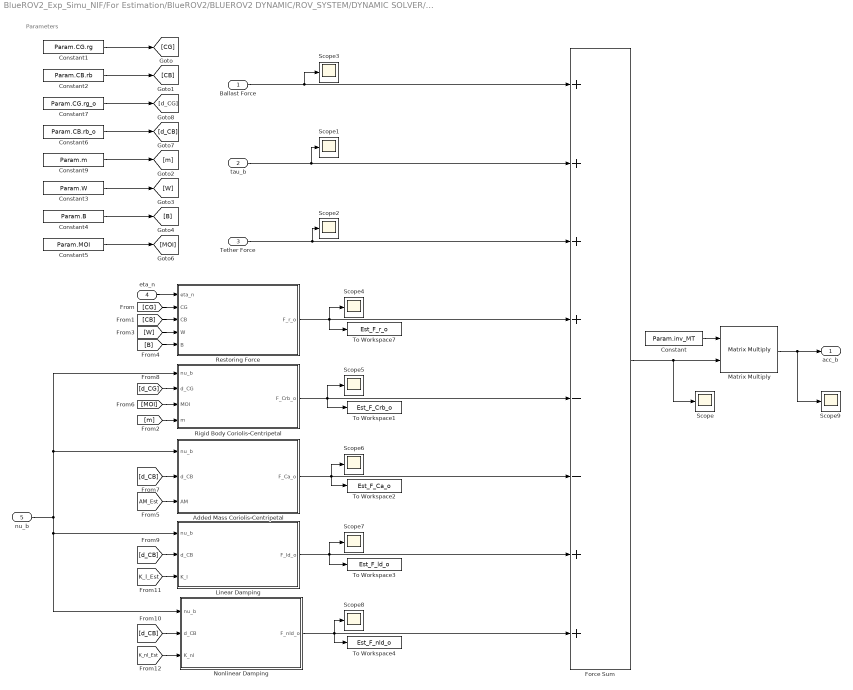
== system BlueROV2_Exp_Simu_NIF/For Estimation/BlueROV2/BLUEROV2 DYNAMIC/ROV_SYSTEM/DYNAMIC SOLVER/BlueROV2_EOM ==
  note: Parameters
  Ballast Force : Inport
  tau_b : Inport  Port=2
  Tether Force : Inport  Port=3
  eta_n : Inport  Port=4
  nu_b : Inport  Port=5
  Added Mass Coriolis-Centripetal : MATLAB Function  TreatAsAtomicUnit=on
  Constant : Constant  Value=Param.inv_MT
  Constant1 : Constant  Value=Param.CG.rg
  Constant2 : Constant  Value=Param.CB.rb
  Constant3 : Constant  Value=Param.W
  Constant4 : Constant  Value=Param.B
  Constant5 : Constant  Value=Param.MOI
  Constant6 : Constant  Value=Param.CB.rb_o
  Constant7 : Constant  Value=Param.CG.rg_o
  Constant9 : Constant  Value=Param.m
  Force Sum : Sum  Inputs=++++--++
  Linear Damping : MATLAB Function  TreatAsAtomicUnit=on
  Matrix Multiply : Product  Multiplication=Matrix(*)
  Nonlinear Damping : MATLAB Function  TreatAsAtomicUnit=on
  Restoring Force : MATLAB Function  TreatAsAtomicUnit=on
  Rigid Body Coriolis-Centripetal : MATLAB Function  TreatAsAtomicUnit=on
  Scope{,1..9} (10 alike) : Scope
  To Workspace1 : ToWorkspace  VariableName=Est_F_Crb_o  SampleTime=-1
  To Workspace2 : ToWorkspace  VariableName=Est_F_Ca_o  SampleTime=-1
  To Workspace3 : ToWorkspace  VariableName=Est_F_ld_o  SampleTime=-1
  To Workspace4 : ToWorkspace  VariableName=Est_F_nld_o  SampleTime=-1
  To Workspace7 : ToWorkspace  VariableName=Est_F_r_o  SampleTime=-1
  acc_b : Outport
  wires:
  eta_n/1 -> Restoring Force/1(eta_n)
  nu_b/1 -> Nonlinear Damping/1(nu_b), Linear Damping/1(nu_b), Rigid Body Coriolis-Centripetal/1(nu_b), Added Mass Coriolis-Centripetal/1(nu_b)
  Force Sum/1 -> Scope/1, Matrix Multiply/2
  Constant/1 -> Matrix Multiply/1
  Matrix Multiply/1 -> Scope9/1, acc_b/1
  Ballast Force/1 -> Scope3/1, Force Sum/1
  tau_b/1 -> Scope1/1, Force Sum/2
  Tether Force/1 -> Scope2/1, Force Sum/3
  Restoring Force/1(F_r_o) -> To Workspace7/1, Force Sum/4, Scope4/1
  Rigid Body Coriolis-Centripetal/1(F_Crb_o) -> Scope5/1, To Workspace1/1, Force Sum/5
  Added Mass Coriolis-Centripetal/1(F_Ca_o) -> To Workspace2/1, Scope6/1, Force Sum/6
  Linear Damping/1(F_ld_o) -> To Workspace3/1, Scope7/1, Force Sum/7
  Nonlinear Damping/1(F_nld_o) -> Scope8/1, To Workspace4/1, Force Sum/8
  Constant1/1 -> [CG]
  Constant2/1 -> [CB]
  Constant6/1 -> [d_CB]
  Constant7/1 -> [d_CG]
  Constant9/1 -> [m]
  Constant3/1 -> [W]
  Constant4/1 -> [B]
  Constant5/1 -> [MOI]
  [CG] -> Restoring Force/2(CG)
  [CB] -> Restoring Force/3(CB)
  [W] -> Restoring Force/4(W)
  [B] -> Restoring Force/5(B)
  [d_CG] -> Rigid Body Coriolis-Centripetal/2(d_CG)
  [m] -> Rigid Body Coriolis-Centripetal/4(m)
  [MOI] -> Rigid Body Coriolis-Centripetal/3(MOI)
  [d_CB] -> Added Mass Coriolis-Centripetal/2(d_CB)
  [AM_Est] -> Added Mass Coriolis-Centripetal/3(AM)
  [d_CB] -> Linear Damping/2(d_CB)
  [d_CB] -> Nonlinear Damping/2(d_CB)
  [K_l_Est] -> Linear Damping/3(K_l)
  [K_nl_Est] -> Nonlinear Damping/3(K_nl)

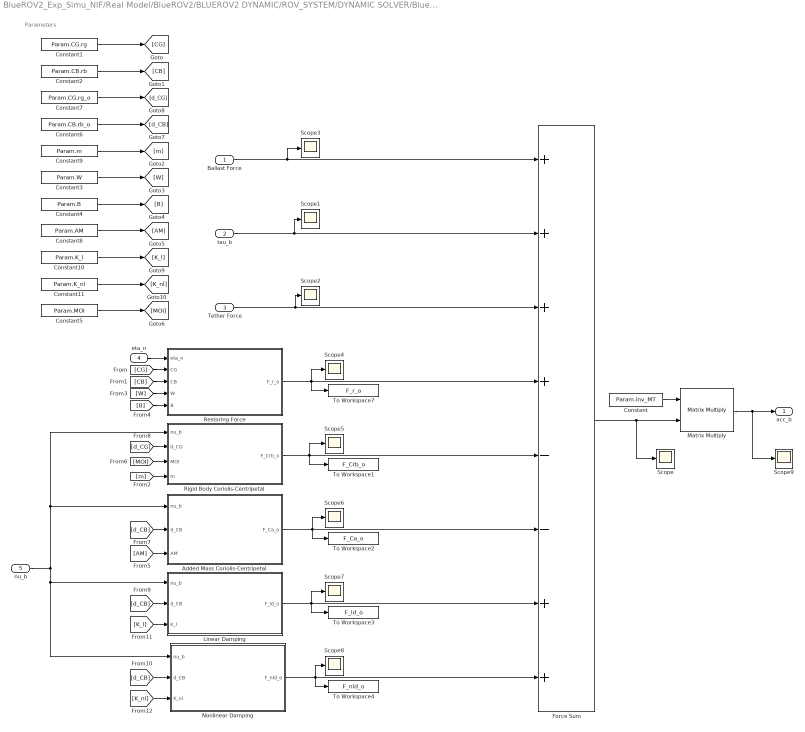
== system BlueROV2_Exp_Simu_NIF/Real Model/BlueROV2/BLUEROV2 DYNAMIC/ROV_SYSTEM/DYNAMIC SOLVER/BlueROV2_EOM ==
  note: Parameters
  Ballast Force : Inport
  tau_b : Inport  Port=2
  Tether Force : Inport  Port=3
  eta_n : Inport  Port=4
  nu_b : Inport  Port=5
  Added Mass Coriolis-Centripetal : MATLAB Function  TreatAsAtomicUnit=on
  Constant : Constant  Value=Param.inv_MT
  Constant1 : Constant  Value=Param.CG.rg
  Constant10 : Constant  Value=Param.K_l
  Constant11 : Constant  Value=Param.K_nl
  Constant2 : Constant  Value=Param.CB.rb
  Constant3 : Constant  Value=Param.W
  Constant4 : Constant  Value=Param.B
  Constant5 : Constant  Value=Param.MOI
  Constant6 : Constant  Value=Param.CB.rb_o
  Constant7 : Constant  Value=Param.CG.rg_o
  Constant8 : Constant  Value=Param.AM
  Constant9 : Constant  Value=Param.m
  Force Sum : Sum  Inputs=++++--++
  Linear Damping : MATLAB Function  TreatAsAtomicUnit=on
  Matrix Multiply : Product  Multiplication=Matrix(*)
  Nonlinear Damping : MATLAB Function  TreatAsAtomicUnit=on
  Restoring Force : MATLAB Function  TreatAsAtomicUnit=on
  Rigid Body Coriolis-Centripetal : MATLAB Function  TreatAsAtomicUnit=on
  Scope{,1..9} (10 alike) : Scope
  To Workspace1 : ToWorkspace  VariableName=F_Crb_o  SampleTime=-1
  To Workspace2 : ToWorkspace  VariableName=F_Ca_o  SampleTime=-1
  To Workspace3 : ToWorkspace  VariableName=F_ld_o  SampleTime=-1
  To Workspace4 : ToWorkspace  VariableName=F_nld_o  SampleTime=-1
  To Workspace7 : ToWorkspace  VariableName=F_r_o  SampleTime=-1
  acc_b : Outport
  wires:
  eta_n/1 -> Restoring Force/1(eta_n)
  nu_b/1 -> Nonlinear Damping/1(nu_b), Linear Damping/1(nu_b), Rigid Body Coriolis-Centripetal/1(nu_b), Added Mass Coriolis-Centripetal/1(nu_b)
  Force Sum/1 -> Scope/1, Matrix Multiply/2
  Constant/1 -> Matrix Multiply/1
  Matrix Multiply/1 -> Scope9/1, acc_b/1
  Ballast Force/1 -> Scope3/1, Force Sum/1
  tau_b/1 -> Scope1/1, Force Sum/2
  Tether Force/1 -> Scope2/1, Force Sum/3
  Restoring Force/1(F_r_o) -> To Workspace7/1, Force Sum/4, Scope4/1
  Rigid Body Coriolis-Centripetal/1(F_Crb_o) -> Scope5/1, To Workspace1/1, Force Sum/5
  Added Mass Coriolis-Centripetal/1(F_Ca_o) -> To Workspace2/1, Scope6/1, Force Sum/6
  Linear Damping/1(F_ld_o) -> To Workspace3/1, Scope7/1, Force Sum/7
  Nonlinear Damping/1(F_nld_o) -> Scope8/1, To Workspace4/1, Force Sum/8
  Constant1/1 -> [CG]
  Constant2/1 -> [CB]
  Constant6/1 -> [d_CB]
  Constant7/1 -> [d_CG]
  Constant9/1 -> [m]
  Constant3/1 -> [W]
  Constant4/1 -> [B]
  Constant8/1 -> [AM]
  Constant5/1 -> [MOI]
  [CG] -> Restoring Force/2(CG)
  [CB] -> Restoring Force/3(CB)
  [W] -> Restoring Force/4(W)
  [B] -> Restoring Force/5(B)
  [d_CG] -> Rigid Body Coriolis-Centripetal/2(d_CG)
  [m] -> Rigid Body Coriolis-Centripetal/4(m)
  [MOI] -> Rigid Body Coriolis-Centripetal/3(MOI)
  [d_CB] -> Added Mass Coriolis-Centripetal/2(d_CB)
  [AM] -> Added Mass Coriolis-Centripetal/3(AM)
  [d_CB] -> Linear Damping/2(d_CB)
  [d_CB] -> Nonlinear Damping/2(d_CB)
  [K_l] -> Linear Damping/3(K_l)
  [K_nl] -> Nonlinear Damping/3(K_nl)
  Constant10/1 -> [K_l]
  Constant11/1 -> [K_nl]

== matlab function BlueROV2_Exp_Simu_NIF/Real Model/Reference Model AGF/Heave/MATLAB Function1 ==
  data: val_checkpoints input; time_stamps input; ref output; t input
function ref = generate_step_signal(val_checkpoints, time_stamps, t)
    % Initialize output signal
    ref = zeros(size(t));

    % Iterate through set points
    for i = 1:length(val_checkpoints)
        value = val_checkpoints(i);
        time = time_stamps(i);

        % Generate step signal
        ref(t >= time) = value;
    end
end

== matlab function BlueROV2_Exp_Simu_NIF/Real Model/Reference Model AGF/Pitch/MATLAB Function1 ==
  data: val_checkpoints input; time_stamps input; ref output; t input
function ref = generate_step_signal(val_checkpoints, time_stamps, t)
    % Initialize output signal
    ref = zeros(size(t));

    % Iterate through set points
    for i = 1:length(val_checkpoints)
        value = val_checkpoints(i);
        time = time_stamps(i);

        % Generate step signal
        ref(t >= time) = value;
    end
end

== matlab function BlueROV2_Exp_Simu_NIF/Real Model/BlueROV2/BLUEROV2 DYNAMIC/ROV_SYSTEM/DYNAMIC SOLVER/BlueROV2_EOM/Restoring Force ==
  data: eta_n input; F_r_o output; CG input; CB input; W input; B input
function F_r_o   = Restoring_Force(eta_n, CG, CB, W, B)
%% Restoring Forces
% Described in Body Frame, at Center of Gravity. ALREADY FOR THE LEFT HAND SIDE
% Orientation
phi = eta_n(4);
theta = eta_n(5);

% Gravity
xg = CG(1);
yg = CG(2);
zg = CG(3);

% Buoyancy
xb = CB(1);
yb = CB(2);
zb = CB(3);

% % Force
% Fg_n = [0; 0; W];
% Fb_n = -[0; 0; B];
% 
% F_r_o = -[Rot_bn(eta_n) * Fg_n + Rot_bn(eta_n) * Fb_n;
%          cross(CG, Rot_bn(eta_n) * Fg_n) + cross(CB, Rot_bn(eta_n) * Fb_n)];

% Force
F_r_o = [(W - B)*sin(theta);
         -(W - B)*cos(theta)*sin(phi);
         -(W - B)*cos(theta)*cos(phi);
         -(yg*W - yb*B)*cos(theta)*cos(phi) + (zg*W - zb*B)*cos(theta)*sin(phi);
         (zg*W - zb*B)*sin(theta) + (xg*W - xb*B)*cos(theta)*cos(phi);
         -(xg*W - xb*B)*cos(theta)*sin(phi) - (yg*W - yb*B)*sin(theta)];

% For debugging
% F_r_o = zeros(6,1);
end

== matlab function BlueROV2_Exp_Simu_NIF/Real Model/Reference Model AGF/Roll/MATLAB Function1 ==
  data: val_checkpoints input; time_stamps input; ref output; t input
function ref = generate_step_signal(val_checkpoints, time_stamps, t)
    % Initialize output signal
    ref = zeros(size(t));

    % Iterate through set points
    for i = 1:length(val_checkpoints)
        value = val_checkpoints(i);
        time = time_stamps(i);

        % Generate step signal
        ref(t >= time) = value;
    end
end

== matlab function BlueROV2_Exp_Simu_NIF/Real Model/Reference Model AGF/Sway/MATLAB Function1 ==
  data: val_checkpoints input; time_stamps input; ref output; t input
function ref = generate_step_signal(val_checkpoints, time_stamps, t)
    % Initialize output signal
    ref = zeros(size(t));

    % Iterate through set points
    for i = 1:length(val_checkpoints)
        value = val_checkpoints(i);
        time = time_stamps(i);

        % Generate step signal
        ref(t >= time) = value;
    end
end

== matlab function BlueROV2_Exp_Simu_NIF/Real Model/Reference Model AGF/Yaw/MATLAB Function1 ==
  data: val_checkpoints input; time_stamps input; ref output; t input
function ref = generate_step_signal(val_checkpoints, time_stamps, t)
    % Initialize output signal
    ref = zeros(size(t));

    % Iterate through set points
    for i = 1:length(val_checkpoints)
        value = val_checkpoints(i);
        time = time_stamps(i);

        % Generate step signal
        ref(t >= time) = value;
    end
end

== matlab function BlueROV2_Exp_Simu_NIF/Real Model/BlueROV2/BLUEROV2 DYNAMIC/ROV_SYSTEM/DYNAMIC SOLVER/BlueROV2_EOM/Rigid Body Coriolis-Centripetal ==
  data: nu_b input; F_Crb_o output; d_CG input; MOI input; m input
function F_Crb_o    = Coriolis_Centripetal_RB_Force(nu_b, d_CG, MOI, m)
%% Coriolis-Centripetal Forces
% Velocity
u = nu_b(1);
v = nu_b(2);
w = nu_b(3);
p = nu_b(4);
q = nu_b(5);
r = nu_b(6);

% Distance from CG to CO
% Defined as d_CG

% Transformed Velocity
V_t_g = H_(-d_CG) * nu_b;  % 6DOF Velocity, expressed in CG

% MOI
Ixx = MOI(1);
Iyy = MOI(2);
Izz = MOI(3);

% CC-Rigid Body
% Described in Body frame, at Center of Gravity

Crb11 = zeros(3); 
Crb12 = [0 m*w -m*v;
         -m*w 0 m*u;
         m*v -m*u 0];
Crb21 = Crb12;
Crb22 = [0 -Izz*r -Iyy*q;
         Izz*r 0 Ixx*p;
         Iyy*q -Ixx*p 0];

Crb = [Crb11 Crb12;
       Crb21 Crb22]; % Rigid Body Coriolis Force Matrix, at Center of Gravity

% Force
F_Crb_o = (H_(d_CG))' * Crb * V_t_g;

% For debugging
% F_Crb_o = Crb * nu_b;
% F_Crb_o = zeros(6,1);
end

== matlab function BlueROV2_Exp_Simu_NIF/Real Model/Reference Model AGF/Continuous/MATLAB Function ==
  data: model_val input; time_val input; y output; t input
function y = generate_step_signal(model_val, time_val, t)
    % Initialize output signal
    y = zeros(size(t));

    % Iterate through set points
    for i = 1:length(model_val)
        value = model_val(i);
        time = time_val(i);

        % Generate step signal
        y(t >= time) = value;
    end
end

== matlab function BlueROV2_Exp_Simu_NIF/Real Model/Reference Model AGF/Surge/MATLAB Function1 ==
  data: val_checkpoints input; time_stamps input; ref output; t input
function ref = generate_step_signal(val_checkpoints, time_stamps, t)
    % Initialize output signal
    ref = zeros(size(t));

    % Iterate through set points
    for i = 1:length(val_checkpoints)
        value = val_checkpoints(i);
        time = time_stamps(i);

        % Generate step signal
        ref(t >= time) = value;
    end
end

== matlab function BlueROV2_Exp_Simu_NIF/Real Model/BlueROV2/BLUEROV2 DYNAMIC/ROV_SYSTEM/DYNAMIC SOLVER/BlueROV2_EOM/Added Mass Coriolis-Centripetal ==
  data: nu_b input; F_Ca_o output; d_CB input; AM input
function F_Ca_o    = Coriolis_Centripetal_AM_Force(nu_b, d_CB, AM)
%% Coriolis-Centripetal Forces
% Velocity
u = nu_b(1);
v = nu_b(2);
w = nu_b(3);
p = nu_b(4);
q = nu_b(5);
r = nu_b(6);

% Distance from CB to CO
% Defined as d_CB

% Transformed Velocity
V_t_b = H_(-d_CB) * nu_b;  % 6DOF Velocity, expressed in CB

% Added Mass Coefficient
Xud = AM(1);
Yvd = AM(2);
Zwd = AM(3);
Kpd = AM(4);
Mqd = AM(5);
Nrd = AM(6);

% CC-Added Mass
% Described in Body frame, at Center of Buoyancy
Ca11 = zeros(3);
Ca12 = [0 -Zwd*w Yvd*v;
        Zwd*w 0 -Xud*u;
        -Yvd*v Xud*u 0];
Ca21 = Ca12;
Ca22 = [0 -Nrd*r Mqd*q;
        Nrd*r 0 -Kpd*p;
        -Mqd*q Kpd*p 0];

Ca = [Ca11 Ca12;
      Ca21 Ca22]; % Added mass Coriolis Force Matrix, at Center of Buoyancy

% Force
F_Ca_o = (H_(d_CB))' * Ca * V_t_b;

% For debugging
% F_Ca_o = Ca * nu_b;
% F_Ca_o = zeros(6,1);
end

== matlab function BlueROV2_Exp_Simu_NIF/Real Model/BlueROV2/BLUEROV2 DYNAMIC/ROV_SYSTEM/DYNAMIC SOLVER/BlueROV2_EOM/Linear Damping ==
  data: F_ld_o output; nu_b input; d_CB input; K_l input
function F_ld_o  = Linear_Damping(nu_b, d_CB, K_l)
% %% Linear Damping Forces
% % Distance from CB to CO
% % Defined as d_CB

% Transformed Velocity
V_t_b = H_(-d_CB) * nu_b;  % 6DOF Velocity, expressed in CB

% Force
F_ld_o = -(H_(d_CB)) * diag(K_l) * V_t_b; 

% For debugging
% F_ld_o = -diag(L_Damping_Matrix) * nu_b; 
% F_ld_o = zeros(6,1); 
end
